simulink model "DYN_6DOF"  (R2018b)
settings: Solver=ode3  StartTime=0.0  StopTime=50  FixedStep=0.01  RelTol=1e-3
(part 1 of 18)
settings Model: Creator=tongn  LastModifiedBy=TMP

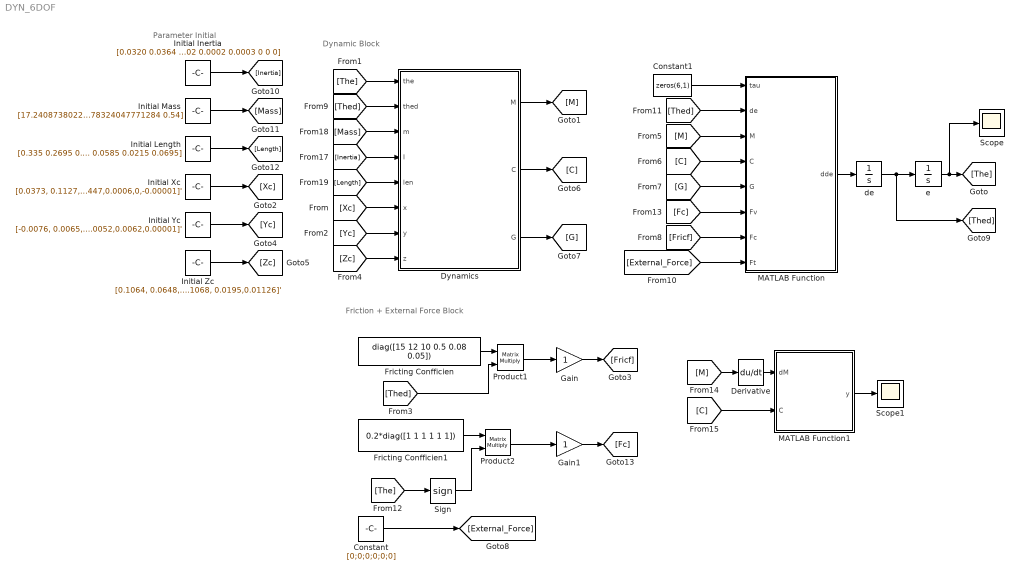
== system DYN_6DOF ==
  note: Parameter Initial
  note: Friction + External Force Block
  note: Dynamic Block
  Constant : Constant  Value=[0;0;0;0;0;0]
  Constant1 : Constant  Value=zeros(6,1)
  Derivative : Derivative
  Dynamics : MATLAB Function  TreatAsAtomicUnit=on
  Fricting Confficien : Constant  Value=diag([15 12 10 0.5 0.08 0.05])
  Fricting Confficien1 : Constant  Value=0.2*diag([1 1 1 1 1 1])
  Gain : Gain
  Gain1 : Gain
  Initial Inertia : Constant  Value=|
      | [0.0320 0.0364 0.0334 0.0017 0.0018 -0.0093;
      | 0.0099, 0.0646, 0.0684, -0.0008, -0.0002, 0.0002; 0.0176, 0.0195, 0.024, -0.001, -0.0002, -0.0007;
      | 0.009 0.0081 0.0037 0 -0.0002 0;
      | 0.0003 0.0002 0.0003 0 0 0;
      | 0.00002 0.0002 0.0003 0 0 0]
  Initial Length : Constant  Value=[0.335 0.2695 0.0905 0.298 0.0585 0.0215 0.0695]
  Initial Mass : Constant  Value=[17.240873802220893 7.3398762571691067 9.1010917011561592 5.3254595389331039 1.2978324047771284 0.54]
  Initial Xc : Constant  Value=[0.0373, 0.1127,0.0447,0.0006,0,-0.00001]'
  Initial Yc : Constant  Value=[-0.0076, 0.0065, 0.0125,0.0052,0.0062,0.00001]'
  Initial Zc : Constant  Value=[0.1064, 0.0648, -0.0554, 0.1068, 0.0195,0.01126]'
  MATLAB Function : MATLAB Function  TreatAsAtomicUnit=on
  MATLAB Function1 : MATLAB Function  TreatAsAtomicUnit=on
  Product1 : Product  Multiplication=Matrix(*)
  Product2 : Product  Multiplication=Matrix(*)
  Scope : Scope
  Scope1 : Scope
  Sign : Signum
  de : Integrator  InitialCondition=zeros(6,1)  IgnoreLimit=on
  e : Integrator  InitialCondition=[0.0001;pi/6;0.0001;0.0001;0.0001;0.0001]  LimitOutput=on  UpperSaturationLimit=[170;90;90;120;60;180]*pi/180  LowerSaturationLimit=-[170;90;90;120;60;180]*pi/180
  wires:
  [Mass] -> Dynamics/3(m)
  Dynamics/2(C) -> [C]
  [Inertia] -> Dynamics/4(I)
  [Thed] -> Product1/2
  [Thed] -> Dynamics/2(thed)
  Product1/1 -> Gain/1
  Fricting Confficien/1 -> Product1/1
  Dynamics/3(G) -> [G]
  Initial Mass/1 -> [Mass]
  [The] -> Dynamics/1(the)
  Initial Length/1 -> [Length]
  [Length] -> Dynamics/5(len)
  Initial Inertia/1 -> [Inertia]
  Dynamics/1(M) -> [M]
  Initial Xc/1 -> [Xc]
  Initial Zc/1 -> [Zc]
  Initial Yc/1 -> [Yc]
  [Xc] -> Dynamics/6(x)
  [Yc] -> Dynamics/7(y)
  [Zc] -> Dynamics/8(z)
  [M] -> MATLAB Function/3(M)
  [C] -> MATLAB Function/4(C)
  [G] -> MATLAB Function/5(G)
  [Fricf] -> MATLAB Function/7(Fc)
  Constant/1 -> [External_Force]
  [External_Force] -> MATLAB Function/8(Ft)
  MATLAB Function/1(dde) -> de/1
  de/1 -> e/1, [Thed]
  e/1 -> Scope/1, [The]
  Constant1/1 -> MATLAB Function/1(tau)
  [Thed] -> MATLAB Function/2(de)
  Fricting Confficien1/1 -> Product2/1
  Product2/1 -> Gain1/1
  [The] -> Sign/1
  Sign/1 -> Product2/2
  [Fc] -> MATLAB Function/6(Fv)
  Gain/1 -> [Fricf]
  Gain1/1 -> [Fc]
  [M] -> Derivative/1
  Derivative/1 -> MATLAB Function1/1(dM)
  [C] -> MATLAB Function1/2(C)
  MATLAB Function1/1(y) -> Scope1/1

== matlab function DYN_6DOF/MATLAB Function ==
  data: tau input; de input; M input; C input; G input; Fv input; Fc input; dde output; Ft input
function dde= fcn(tau,de,M,C,G,Fv,Fc,Ft)
J = zeros(6);

dde = inv(M)*(tau - C*de - G - Fv - Fc - transpose(J)*Ft);
